simulink model "model_simulate"  (R2020a)
settings: Solver=VariableStepAuto  StartTime=0.0  StopTime=10.0  RelTol=1e-3
settings Model: Creator=jorda  LastModifiedBy=jorda

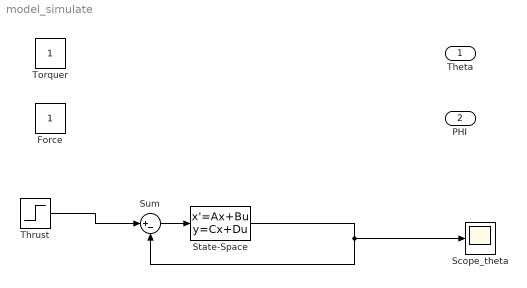
== system model_simulate ==
  Force : Constant
  Scope_theta : Scope
  State-Space : StateSpace  InitialCondition=0
  Sum : Sum  Inputs=|+-
  Thrust : Step  SampleTime=0
  Torquer : Constant
  Theta : Outport
  PHI : Outport  Port=2
  wires:
  Thrust/1 -> Sum/1
  Sum/1 -> State-Space/1
  State-Space/1 -> Sum/2, Scope_theta/1
